simulink library "Power_Shaft4_Electric_L1_R1_L2_R2"  (R2025b)
settings: Solver=VariableStepAuto  StartTime=0.0  StopTime=10.0  RelTol=1e-3
values from neighbouring files (symbols this model uses):
  VDatabase = evalin('base','VDatabase')    [sm_car_controlparam_Ideal_L1_R1_L2_R2_achilles.m]    (also in sm_car_controlparam_Ideal_L1_R1_L2_R2_default.m)
undefined symbols (not defined in the file or in its folder): ShaftL1, ShaftL2, ShaftR1, ShaftR2
libraries: Power_Components x5, fl_lib x2, sm_lib x1, Cooling_Motor4 x1
Description:
  | Component of Simscape Vehicle Templates Library
  | 
  | Copyright 2018-2025 The MathWorks, Inc.
settings Model: Creator=smiller  LastModifiedBy=smiller
settings SolverCC: AlgebraicLoopSolver=TrustRegion
settings DataIOCC: ReturnWorkspaceOutputs=off
settings OptimizationCC: ReuseModelBlockBuffer=off
settings DebuggingCC: UnconnectedInputMsg=warning  UnconnectedOutputMsg=warning  UnconnectedLineMsg=warning  ArithmeticOperatorsInVariantConditions=warning
settings ModelReferenceCC: EnableRefExpFcnMdlSchedulingChecks=on
settings SFSimCC: CustomCodeUndefinedFunction=UseInterfaceOnly
settings RTWCC: GPUComputeCapability=3.5

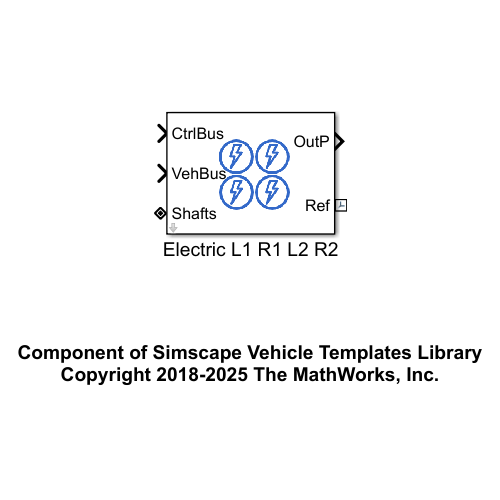
[thumbnail: Simulink's stored preview of the top-level diagram]
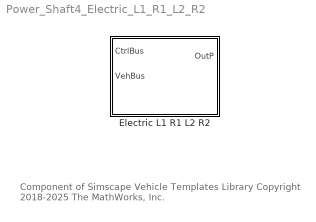
== system Power_Shaft4_Electric_L1_R1_L2_R2 ==
  note: Component of Simscape Vehicle Templates Library
      | Copyright 2018-2025 The MathWorks, Inc.
  Electric L1 R1 L2 R2 : Subsystem  mask(Electric Propulsion with Four Motors){Power=VDatabase.Power.Electric3Motor_A1_L2_R2_default}
      mask prompts: Power "Power 4 Motor (structure)"
      mask help: Four electric motors with optional cooling system. Physical connections for the four motor shafts are in bus Shafts.
      mask Display: image('sm_car_vehicle_power_e4motor_IMAGE.png');

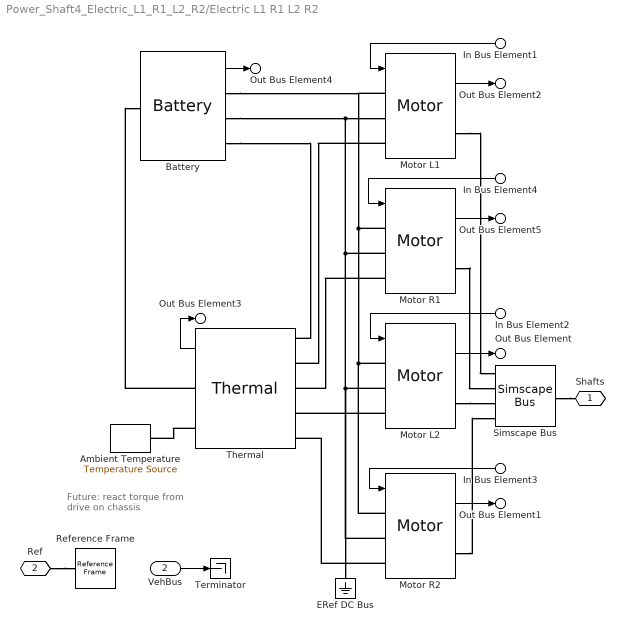
== system Power_Shaft4_Electric_L1_R1_L2_R2/Electric L1 R1 L2 R2 ==
  note: Future:
      | react torque
      | from drive
      | on chassis
  In Bus Element1 : Inport  PortName=CtrlBus  Element=MMotorL1Demand
  In Bus Element2 : Inport  PortName=CtrlBus  Element=MMotorL2Demand
  In Bus Element3 : Inport  PortName=CtrlBus  Element=MMotorR2Demand
  In Bus Element4 : Inport  PortName=CtrlBus  Element=MMotorR1Demand
  VehBus : Inport  Port=2
  Ambient Temperature : fl_lib/Thermal/Thermal Sources/Temperature Source  temperature=Power.TAmbient.Value K
  Battery : Power_Components/Battery  SystemSampleTime=-1  VariantActivationTime=update diagram  EmptyChoice=off  PassThrough=off  PassThroughVariantControl=(default)  EmptyChoiceVariantControl=(default)  AllowFlexibleInterface=on  Latency=0  AutoFrameSizeCalculation=off
  ERef DC Bus : fl_lib/Electrical/Electrical Elements/Electrical Reference
  Motor L1 : Power_Components/Motor  Motor=Power.MotorL1
  Motor L2 : Power_Components/Motor  Motor=Power.MotorL2
  Motor R1 : Power_Components/Motor  Motor=Power.MotorL1
  Motor R2 : Power_Components/Motor  Motor=Power.MotorL2
  Reference Frame : sm_lib/Frames and Transforms/Reference Frame
  Simscape Bus : SimscapeBus  HierarchyStrings=ShaftL1;ShaftR1;ShaftL2;ShaftR2
  Terminator : Terminator
  Thermal : Cooling_Motor4/Thermal  VariantControl=Variant1  LabelModeActiveChoice=Liquid_Loop1  VariantLabel=Power.Cooling.class.Value
      settings: AttributesFormatString=%<ActiveVariant>
  Shafts : PMIOPort  Side=Left
  Ref : PMIOPort  Port=2  Side=Right
  Out Bus Element : Outport  VectorParamsAs1DForOutWhenUnconnected=off  PortName=OutP  Element=MotorL2
  Out Bus Element1 : Outport  VectorParamsAs1DForOutWhenUnconnected=off  PortName=OutP  Element=MotorR2
  Out Bus Element2 : Outport  VectorParamsAs1DForOutWhenUnconnected=off  PortName=OutP  Element=MotorL1
  Out Bus Element3 : Outport  VectorParamsAs1DForOutWhenUnconnected=off  PortName=OutP  Element=Thermal
  Out Bus Element4 : Outport  VectorParamsAs1DForOutWhenUnconnected=off  PortName=OutP  Element=Battery
  Out Bus Element5 : Outport  VectorParamsAs1DForOutWhenUnconnected=off  PortName=OutP  Element=MotorR1
  wires:
  In Bus Element2/1 -> Motor L2/1
  In Bus Element1/1 -> Motor L1/1
  Motor L2/1 -> Out Bus Element/1
  Motor R2/1 -> Out Bus Element1/1
  Motor L1/1 -> Out Bus Element2/1
  In Bus Element3/1 -> Motor R2/1
  Thermal/1 -> Out Bus Element3/1
  VehBus/1 -> Terminator/1
  Battery/1 -> Out Bus Element4/1
  Motor R1/1 -> Out Bus Element5/1
  In Bus Element4/1 -> Motor R1/1
  connections:
  Motor R2/RConn1 -- Simscape Bus/LConn4
  Motor L2/LConn2 -- Motor R2/LConn2 -- ERef DC Bus/LConn1 -- Motor R1/LConn2 -- Battery/RConn2 -- Motor L1/LConn2
  Motor L2/LConn1 -- Motor R1/LConn1 -- Battery/RConn1 -- Motor L1/LConn1 -- Motor R2/LConn1
  Motor L1/RConn1 -- Simscape Bus/LConn1
  Motor L2/RConn1 -- Simscape Bus/LConn3
  Simscape Bus/RConn1 -- Shafts/RConn1
  Ref/RConn1 -- Reference Frame/RConn1
  Motor L1/LConn3 -- Thermal/LConn2
  Motor L2/LConn3 -- Thermal/LConn4
  Motor R2/LConn3 -- Thermal/LConn5
  Thermal/RConn2 -- Ambient Temperature/LConn1
  Battery/RConn3 -- Thermal/LConn1
  Thermal/RConn1 -- Battery/LConn1
  Motor R1/RConn1 -- Simscape Bus/LConn2
  Motor R1/LConn3 -- Thermal/LConn3
